simulink model "adaptiveBS"  (R2022a)
settings: Solver=VariableStepAuto  StartTime=0.0  StopTime=timeSpan  RelTol=1e-4
values from neighbouring files (symbols this model uses):
  K_d = 100 * eye(n)    [adaptiveBS_main.m]
  Lambda = 1 * eye(n)    [adaptiveBS_main.m]
  max_tau = 100 * [1 1 1 1 1 1]    [adaptiveBS_main.m]
  R = 10 * eye(n * 10)    [adaptiveBS_main.m]
undefined symbols (not defined in the file or in its folder): pi_est_0, pi_real
(part 5 of 5)

== matlab function adaptiveBS/Adattamento/MATLAB Function1 ==
  data: q input; Y output; dq input; ddq input
function Y = regressor(q, dq, ddq)

    % https://github.com/cdsousa/SymPyBotics

    %% Denavit-Hartenberg
    a2 = 0.4318;    a3 = 0.0203;
    d3 = 0.15005;   d4 = 0.4318;

    %% Variabili di giunto
    % q1 = q(1);  dq1 = dq(1);   ddq1 = ddq(1);
    % q2 = q(2);  dq2 = dq(2);   ddq2 = ddq(2);
    % q3 = q(3);  dq3 = dq(3);   ddq3 = ddq(3);
    % q4 = q(4);  dq4 = dq(4);   ddq4 = ddq(4);
    % q5 = q(5);  dq5 = dq(5);   ddq5 = ddq(5);
    % q6 = q(6);  dq6 = dq(6);   ddq6 = ddq(6);

    %% parms
    % (L_1xx, L_1xy, L_1xz, L_1yy, L_1yz, L_1zz, l_1x, l_1y, l_1z, m_1, L_2xx, L_2xy, L_2xz, L_2yy, L_2yz, L_2zz, l_2x, l_2y, l_2z, m_2, L_3xx, L_3xy, L_3xz, L_3yy, L_3yz, L_3zz, l_3x, l_3y, l_3z, m_3, L_4xx, L_4xy, L_4xz, L_4yy, L_4yz, L_4zz, l_4x, l_4y, l_4z, m_4, L_5xx, L_5xy, L_5xz, L_5yy, L_5yz, L_5zz, l_5x, l_5y, l_5z, m_5, L_6xx, L_6xy, L_6xz, L_6yy, L_6yz, L_6zz, l_6x, l_6y, l_6z, m_6)
    % Where:
    %   L is the link inertia tensor computed about the link frame;
    %   l is the link first moment of inertia;
    %   m is the link mass.
    % These are the so-called barycentric parameters, with respect to which the dynamic model is linear.


    x0 = sin(q(2));
    x1 = cos(q(2));
    x2 = dq(1) * x1;
    x3 = dq(2) * x2;
    x4 = ddq(1) * x0 + x3;
    x5 = dq(1) * x0;
    x6 = dq(2) * x5;
    x7 = -dq(2);
    x8 = x5 * x7;
    x9 = ddq(1) * x1;
    x10 = x8 + x9;
    x11 = x1 * (x3 + x4);
    x12 = ((dq(2)) * (dq(2)));
    x13 = ((x5) * (x5));
    x14 = -x13;
    x15 = x2 * x5;
    x16 = ddq(2) + x15;
    x17 = -x3;
    x18 = ((x2) * (x2));
    x19 = -x12;
    x20 = -x15;
    x21 = -a2;
    x22 = ((x0) * (x0)) * x21 + ((x1) * (x1)) * x21;
    x23 = a2 * dq(2);
    x24 = x23 * x5;
    x25 = x22 * x9 + x24;
    x26 = -x25;
    x27 = x24 + x25;
    x28 = -x18;
    x29 = x2 * x22;
    x30 = 9.81 * x0;
    x31 = a2 * ddq(2) + 9.81 * x1;
    x32 = sin(q(3));
    x33 = x10 * x32;
    x34 = cos(q(3));
    x35 = x34 * x4;
    x36 = x2 * x34;
    x37 = -x32;
    x38 = x37 * x5;
    x39 = x36 + x38;
    x40 = -dq(3);
    x41 = -x40;
    x42 = x33 + x35 + x39 * x41;
    x43 = x2 * x32;
    x44 = x34 * x5;
    x45 = x43 + x44;
    x46 = -x45;
    x47 = x40 + x7;
    x48 = x46 * x47;
    x49 = -ddq(2) - ddq(3);
    x50 = x39 * x45;
    x51 = -x50;
    x52 = x49 + x51;
    x53 = ((x45) * (x45));
    x54 = ((x47) * (x47));
    x55 = -x54;
    x56 = x53 + x55;
    x57 = x45 * x47;
    x58 = x10 * x34;
    x59 = x37 * x4;
    x60 = x40 * x45 + x58 + x59;
    x61 = x57 + x60;
    x62 = x34 * x61;
    x63 = x39 * x47;
    x64 = -x63;
    x65 = x42 + x64;
    x66 = x49 + x50;
    x67 = ((x39) * (x39));
    x68 = -x67;
    x69 = x54 + x68;
    x70 = x34 * x66;
    x71 = x55 + x68;
    x72 = -d3;
    x73 = x32 * x72;
    x74 = a3 * ((x32) * (x32)) + a3 * ((x34) * (x34));
    x75 = x37 * x74;
    x76 = dq(2) * x74 + x23 * x34 + x43 * x72 + x44 * x72;
    x77 = a3 * dq(3);
    x78 = x76 + x77;
    x79 = x26 + x46 * x77 + x58 * x74 + x59 * x74;
    x80 = d3 * x36 + x23 * x32;
    x81 = d3 * x38 + x80;
    x82 = x39 * x81;
    x83 = x46 * x78 + x79 + x82;
    x84 = x37 * x83;
    x85 = -x49;
    x86 = x50 + x85;
    x87 = x34 * x86;
    x88 = x1 * x22;
    x89 = x34 * x83;
    x90 = -x53;
    x91 = x68 + x90;
    x92 = x34 * x74;
    x93 = -x29;
    x94 = x36 * x74 + x38 * x74 + x93;
    x95 = x39 * x94;
    x96 = x47 * x78;
    x97 = d3 * x58 + x30 * x34 + x31 * x32 + x4 * x73 + x41 * x76 + x7 * x77;
    x98 = x95 - x96 - x97;
    x99 = x57 - x60;
    x100 = x42 + x63;
    x101 = a3 * ddq(3) + ddq(2) * x74 + x30 * x37 + x31 * x34 + x33 * x72 + x35 * x72 + x40 * (x5 * x73 + x80);
    x102 = x47 * x81;
    x103 = x101 - x102 + x45 * x94;
    x104 = x103 * x34;
    x105 = x100 * x34;
    x106 = x45 * x78 - x79 - x82;
    x107 = x55 + x90;
    x108 = -x42 + x63;
    x109 = x107 * x34;
    x110 = -x95 + x96 + x97;
    x111 = cos(q(4));
    x112 = sin(q(4));
    x113 = x112 * x49;
    x114 = x111 * x42;
    x115 = x112 * x45;
    x116 = x111 * x47;
    x117 = x115 - x116;
    x118 = -dq(4);
    x119 = x113 + x114 + x117 * x118;
    x120 = x112 * x47;
    x121 = x111 * x45;
    x122 = x120 + x121;
    x123 = dq(4) + x39;
    x124 = x122 * x123;
    x125 = -x124;
    x126 = x111 * x119 + x112 * x125;
    x127 = x117 * x122;
    x128 = x117 * x123;
    x129 = x119 + x128;
    x130 = ((x123) * (x123));
    x131 = -x130;
    x132 = ((x122) * (x122));
    x133 = x131 + x132;
    x134 = -x117;
    x135 = x122 * x134;
    x136 = ddq(4) + x60;
    x137 = x135 + x136;
    x138 = x111 * x137 + x112 * x133;
    x139 = -x111;
    x140 = x112 * x42;
    x141 = dq(4) * x122 + x139 * x49 + x140;
    x142 = x124 + x141;
    x143 = x123 * x134;
    x144 = x119 + x143;
    x145 = x111 * x142 + x112 * x144;
    x146 = -x132;
    x147 = ((x117) * (x117));
    x148 = x146 + x147;
    x149 = x111 * x143 + x112 * x124;
    x150 = x127 + x136;
    x151 = x112 * x150;
    x152 = -x147;
    x153 = x130 + x152;
    x154 = x111 * x153 + x151;
    x155 = x125 + x141;
    x156 = x111 * x128 + x112 * x141;
    x157 = x127 - x136;
    x158 = d4 * x111;
    x159 = -d4;
    x160 = d4 * x116 + x111 * x81 + x112 * x94 + x115 * x159;
    x161 = d4 * x120 + d4 * x121 + x112 * x81 + x139 * x94;
    x162 = -x161;
    x163 = x101 + x117 * x160 + x122 * x162;
    x164 = x131 + x152;
    x165 = x112 * x164;
    x166 = x112 * x163 + x157 * x158 + x159 * x165;
    x167 = x142 * x34;
    x168 = x139 * x157 + x165;
    x169 = x112 * x157;
    x170 = x111 * x164 + x169;
    x171 = x123 * x160;
    x172 = x122 * x78;
    x173 = d4 * x113 + d4 * x114 + dq(4) * x160 + x112 * x97 + x139 * x79;
    x174 = -x173;
    x175 = x171 - x172 + x174;
    x176 = -x141;
    x177 = x124 + x176;
    x178 = x112 * x177;
    x179 = x129 * x139 + x178;
    x180 = x146 + x152;
    x181 = x180 * x34;
    x182 = x112 * x129;
    x183 = x111 * x177 + x182;
    x184 = x111 * x97 + x112 * x79 + x118 * x161 + x140 * x159 + x158 * x49;
    x185 = x117 * x78 + x123 * x162 - x184;
    x186 = -x171 + x172 + x173;
    x187 = x111 * x186 + x112 * x185 + x129 * x158 + x159 * x178;
    x188 = x131 + x146;
    x189 = x139 * x188 + x151;
    x190 = -x119 + x128;
    x191 = x190 * x34;
    x192 = x123 * x161 + x134 * x78 + x184;
    x193 = x112 * x188;
    x194 = x111 * x150 + x193;
    x195 = -x101;
    x196 = x122 * x161 + x134 * x160 + x195;
    x197 = x111 * x196 + x151 * x159 + x158 * x188;
    x198 = x112 * x192;
    x199 = x139 * x186 + x198;
    x200 = x112 * x186;
    x201 = x111 * x192 + x200;
    x202 = x158 * x186 + x159 * x198;
    x203 = x163 * x34;
    x204 = sin(q(5));
    x205 = cos(q(5));
    x206 = x122 * x205 + x123 * x204;
    x207 = -dq(5);
    x208 = x134 + x207;
    x209 = x206 * x208;
    x210 = -x209;
    x211 = -x204;
    x212 = x122 * x211 + x123 * x205;
    x213 = -x207;
    x214 = x119 * x205 + x136 * x204 + x212 * x213;
    x215 = x204 * x214 + x205 * x210;
    x216 = x205 * x214 + x210 * x211;
    x217 = x206 * x212;
    x218 = -x217;
    x219 = x111 * x216 + x112 * x218;
    x220 = x208 * x212;
    x221 = x214 + x220;
    x222 = -x221;
    x223 = -ddq(5) + x176;
    x224 = x218 + x223;
    x225 = ((x206) * (x206));
    x226 = ((x208) * (x208));
    x227 = -x226;
    x228 = x225 + x227;
    x229 = x205 * x224 + x211 * x228;
    x230 = x111 * x229 + x112 * x222;
    x231 = x204 * x224 + x205 * x228;
    x232 = -x225;
    x233 = ((x212) * (x212));
    x234 = -x232 - x233;
    x235 = -x220;
    x236 = x214 + x235;
    x237 = x119 * x211 + x136 * x205 + x206 * x207;
    x238 = x209 + x237;
    x239 = x205 * x238 + x211 * x236;
    x240 = x111 * x239 + x112 * x234;
    x241 = x204 * x238 + x205 * x236;
    x242 = -x223;
    x243 = x205 * x235 + x209 * x211;
    x244 = x111 * x243 + x112 * x242;
    x245 = x204 * x235 + x205 * x209;
    x246 = x217 + x223;
    x247 = -x233;
    x248 = x226 + x247;
    x249 = x205 * x248 + x211 * x246;
    x250 = -x210 - x237;
    x251 = x111 * x249 + x112 * x250;
    x252 = x205 * x246;
    x253 = x204 * x248 + x252;
    x254 = x204 * x220 + x205 * x237;
    x255 = x205 * x220 + x211 * x237;
    x256 = -x218;
    x257 = x111 * x255 + x112 * x256;
    x258 = -x238;
    x259 = x112 * x258;
    x260 = x217 + x242;
    x261 = x227 + x247;
    x262 = x205 * x261 + x211 * x260;
    x263 = x111 * x262 + x259;
    x264 = x204 * x261 + x205 * x260;
    x265 = x264 * x34;
    x266 = -x206;
    x267 = x160 * x211 + x205 * x78;
    x268 = x160 * x205 + x204 * x78;
    x269 = x212 * x268;
    x270 = x174 + x266 * x267 + x269;
    x271 = x205 * x270;
    x272 = x211 * x270;
    x273 = x112 * x262;
    x274 = x208 * x268;
    x275 = x101 * x205 + x184 * x211 + x207 * x268;
    x276 = -x275;
    x277 = -x162 * x266 - x274 - x276;
    x278 = x111 * x272 + x112 * x277 + x158 * x258 + x159 * x273;
    x279 = x139 * x258 + x273;
    x280 = x209 - x237;
    x281 = x205 * x280 + x211 * x221;
    x282 = x112 * x281;
    x283 = -x232 - x247;
    x284 = x139 * x283 + x282;
    x285 = x162 * x206 - x274 + x275;
    x286 = x205 * x285;
    x287 = x162 * x212;
    x288 = x208 * x267;
    x289 = x101 * x204 + x184 * x205 + x213 * x267;
    x290 = x287 - x288 - x289;
    x291 = x211 * x290 + x286;
    x292 = x111 * x291 + x158 * x283 + x159 * x282;
    x293 = x204 * x285 + x205 * x290;
    x294 = x204 * x280 + x205 * x221;
    x295 = x294 * x34;
    x296 = x112 * x283;
    x297 = x111 * x281 + x296;
    x298 = x227 + x232;
    x299 = x204 * x246 + x205 * x298;
    x300 = x299 * x34;
    x301 = -x287 + x288 + x289;
    x302 = -x301;
    x303 = x211 * x298 + x252;
    x304 = x112 * x303;
    x305 = x214 - x220;
    x306 = -x174 + x206 * x267 - x269;
    x307 = x205 * x306;
    x308 = x111 * x307 + x112 * x302 + x158 * x305 + x159 * x304;
    x309 = x139 * x305 + x304;
    x310 = x204 * x306;
    x311 = x112 * x305;
    x312 = x111 * x303 + x311;
    x313 = x205 * x301 + x211 * x285;
    x314 = x112 * x313;
    x315 = -x270;
    x316 = x158 * x315 + x159 * x314;
    x317 = x139 * x315 + x314;
    x318 = x112 * x315;
    x319 = x111 * x313 + x318;
    x320 = x204 * x301 + x286;
    x321 = x320 * x34;
    x322 = sin(q(6));
    x323 = cos(q(6));
    x324 = x206 * x323 + x208 * x322;
    x325 = dq(6) + x212;
    x326 = x324 * x325;
    x327 = -x322;
    x328 = x206 * x327 + x208 * x323;
    x329 = dq(6) * x328 + x214 * x323 + x223 * x322;
    x330 = x323 * x329 + x326 * x327;
    x331 = x324 * x328;
    x332 = -x331;
    x333 = x205 * x330 + x211 * x332;
    x334 = -x322 * x329 - x323 * x326;
    x335 = x111 * x333 + x112 * x334;
    x336 = x204 * x330 + x205 * x332;
    x337 = x325 * x328;
    x338 = x329 + x337;
    x339 = -x326;
    x340 = -dq(6);
    x341 = x214 * x327 + x223 * x323 + x324 * x340;
    x342 = x339 + x341;
    x343 = x323 * x342 + x327 * x338;
    x344 = ((x328) * (x328));
    x345 = -x344;
    x346 = ((x324) * (x324));
    x347 = x345 + x346;
    x348 = x204 * x343 + x205 * x347;
    x349 = x205 * x343 + x211 * x347;
    x350 = -x322 * x342 - x323 * x338;
    x351 = x111 * x349 + x112 * x350;
    x352 = -x337;
    x353 = x329 + x352;
    x354 = ((x325) * (x325));
    x355 = -x346;
    x356 = x354 + x355;
    x357 = ddq(6) + x237;
    x358 = x331 + x357;
    x359 = x323 * x358;
    x360 = x327 * x356 + x359;
    x361 = x204 * x360 + x205 * x353;
    x362 = x205 * x360 + x211 * x353;
    x363 = -x322 * x358 - x323 * x356;
    x364 = x111 * x362 + x112 * x363;
    x365 = x323 * x352 + x327 * x341;
    x366 = x205 * x365 + x211 * x331;
    x367 = -x322 * x352 - x323 * x341;
    x368 = x111 * x366 + x112 * x367;
    x369 = x204 * x365 + x205 * x331;
    x370 = x326 + x341;
    x371 = -x354;
    x372 = x344 + x371;
    x373 = x332 + x357;
    x374 = x323 * x372 + x327 * x373;
    x375 = x205 * x374 + x211 * x370;
    x376 = -x322 * x372 - x323 * x373;
    x377 = x111 * x375 + x112 * x376;
    x378 = x204 * x374 + x205 * x370;
    x379 = x323 * x337 + x327 * x339;
    x380 = x204 * x379 + x205 * x357;
    x381 = x205 * x379 + x211 * x357;
    x382 = -x322 * x337 - x323 * x339;
    x383 = x111 * x381 + x112 * x382;
    x384 = x345 + x371;
    x385 = x323 * x384 + x327 * x358;
    x386 = x326 - x341;
    x387 = x204 * x385 + x205 * x386;
    x388 = x34 * x387;
    x389 = -x322 * x384 - x359;
    x390 = x205 * x385 + x211 * x386;
    x391 = x112 * x390;
    x392 = -x324;
    x393 = x162 * x323 + x268 * x327;
    x394 = x162 * x322 + x268 * x323;
    x395 = x328 * x394;
    x396 = x276 + x392 * x393 + x395;
    x397 = -x323 * x396;
    x398 = x174 * x323 + x289 * x327 + x340 * x394;
    x399 = x325 * x394;
    x400 = x267 * x392 + x398 + x399;
    x401 = x327 * x396;
    x402 = x205 * x401 + x211 * x400;
    x403 = x111 * x402 + x112 * x397 + x158 * x389 + x159 * x391;
    x404 = x139 * x389 + x391;
    x405 = x112 * x389;
    x406 = x111 * x390 + x405;
    x407 = x204 * x401 + x205 * x400;
    x408 = x325 * x393;
    x409 = x267 * x328;
    x410 = dq(6) * x393 + x174 * x322 + x289 * x323;
    x411 = x408 - x409 - x410;
    x412 = x275 + x324 * x393 - x395;
    x413 = x323 * x412;
    x414 = x204 * x413 + x205 * x411;
    x415 = x355 + x371;
    x416 = x331 - x357;
    x417 = x323 * x416 + x327 * x415;
    x418 = x204 * x417 + x205 * x338;
    x419 = -x322 * x416 - x323 * x415;
    x420 = x112 * x419;
    x421 = x205 * x417 + x211 * x338;
    x422 = x111 * x421 + x420;
    x423 = x112 * x421;
    x424 = x139 * x419 + x423;
    x425 = -x322 * x412;
    x426 = x205 * x413 + x211 * x411;
    x427 = x111 * x426 + x112 * x425 + x158 * x419 + x159 * x423;
    x428 = x34 * x418;
    x429 = -x329 + x337;
    x430 = -x322 * x370 - x323 * x429;
    x431 = x345 + x355;
    x432 = x323 * x370 + x327 * x429;
    x433 = x205 * x432 + x211 * x431;
    x434 = x112 * x433;
    x435 = x139 * x430 + x434;
    x436 = x267 * x324 - x398 - x399;
    x437 = -x408 + x409 + x410;
    x438 = x323 * x437;
    x439 = -x322 * x436 - x438;
    x440 = x323 * x436 + x327 * x437;
    x441 = x205 * x440;
    x442 = x111 * x441 + x112 * x439 + x158 * x430 + x159 * x434;
    x443 = x204 * x432 + x205 * x431;
    x444 = x112 * x430;
    x445 = x111 * x433 + x444;
    x446 = x204 * x440;
    x447 = x34 * x443;
    x448 = -x322 * x437 - x323 * x400;
    x449 = x327 * x400 + x438;
    x450 = x205 * x449 + x211 * x412;
    x451 = x112 * x450;
    x452 = x158 * x448 + x159 * x451;
    x453 = x204 * x449 + x205 * x412;
    x454 = x139 * x448 + x451;
    x455 = x112 * x448;
    x456 = x111 * x450 + x455;
    x457 = x34 * x453;
    x458 = x31 + x5 * x93;
    x459 = -x100;
    x460 = -x67 - x90;
    x461 = -x48 - x60;
    x462 = -x51;
    x463 = -x102 - x195 - x46 * x94;
    x464 = -x110;
    x465 = -x112 * x119 - x125 * x139;
    x466 = -x112 * x137 - x133 * x139;
    x467 = -x112 * x142 - x139 * x144;
    x468 = -x112 * x143 - x124 * x139;
    x469 = -x112 * x153 - x139 * x150;
    x470 = -x112 * x128 - x139 * x141;
    x471 = -d4 * x169 - x139 * x163 - x158 * x164;
    x472 = -d4 * x182 - x139 * x185 - x158 * x177 - x200;
    x473 = -d4 * x193 - x112 * x196 - x150 * x158;
    x474 = -d4 * x200 - x158 * x192;
    x475 = -x112 * x216 - x139 * x218;
    x476 = -x112 * x229 - x139 * x222;
    x477 = -x112 * x239 - x139 * x234;
    x478 = -x112 * x243 - x139 * x242;
    x479 = -x112 * x249 - x139 * x250;
    x480 = -x112 * x255 - x139 * x256;
    x481 = -d4 * x259 - x112 * x272 - x139 * x277 - x158 * x262;
    x482 = -d4 * x296 - x112 * x291 - x158 * x281;
    x483 = -d4 * x311 - x112 * x307 - x139 * x302 - x158 * x303;
    x484 = -d4 * x318 - x158 * x313;
    x485 = -x112 * x333 - x139 * x334;
    x486 = -x112 * x349 - x139 * x350;
    x487 = -x112 * x362 - x139 * x363;
    x488 = -x112 * x366 - x139 * x367;
    x489 = -x112 * x375 - x139 * x376;
    x490 = -x112 * x381 - x139 * x382;
    x491 = -d4 * x405 - x112 * x402 - x139 * x397 - x158 * x390;
    x492 = -d4 * x420 - x112 * x426 - x139 * x425 - x158 * x421;
    x493 = -d4 * x444 - x112 * x441 - x139 * x439 - x158 * x433;
    x494 = -d4 * x455 - x158 * x450;

    
    n = 6;
    H = zeros(n * n * 10, 1); % = 360       Y = 6 * 60

    H(1) = 0;
    H(2) = 0;
    H(3) = 0;
    H(4) = ddq(1);
    H(5) = 0;
    H(6) = 0;
    H(7) = 0;
    H(8) = 0;
    H(9) = 0;
    H(10) = 0;
    H(11) = x0 * x4 + x1 * x6;
    H(12) = x0 * (x10 + x8) + x11;
    H(13) = x0 * x16 + x1 * (x12 + x14);
    H(14) = x0 * x17 + x1 * x10;
    H(15) = x0 * (x18 + x19) + x1 * (ddq(2) + x20);
    H(16) = x0 * x3 + x1 * x8;
    H(17) = x1 * x22 * (-x10 + x6) + x1 * (-x24 + x26);
    H(18) = x0 * x27 + x11 * x22;
    H(19) = x0 * (x29 * x5 - x31) + x1 * x22 * (x14 + x28) + x1 * (x2 * x29 + x23 * x7 + x30);
    H(20) = x1 * x22 * x27;
    H(21) = x0 * (x34 * x42 + x37 * x48) + x1 * (x32 * x42 + x34 * x48);
    H(22) = x0 * (x34 * x52 + x37 * x56) + x1 * (x32 * x52 + x34 * x56);
    H(23) = x0 * (x37 * x65 + x62) + x1 * (x32 * x61 + x34 * x65);
    H(24) = x0 * (x34 * x64 + x37 * x57) + x1 * (x32 * x64 + x34 * x57);
    H(25) = x0 * (x34 * x69 + x37 * x66) + x1 * (x32 * x69 + x70);
    H(26) = x0 * (x34 * x63 + x37 * x60) + x1 * (x32 * x63 + x34 * x60);
    H(27) = x0 * (x61 * x75 + x71 * x73 + x72 * x87 + x84) + x1 * (d3 * x34 * x71 + x62 * x74 + x73 * x86 + x89) - x61 * x88;
    H(28) = x0 * (x104 + x105 * x72 + x37 * x98 + x73 * x99 + x75 * x91) + x1 * (d3 * x34 * x99 + x100 * x73 + x103 * x32 + x34 * x98 + x91 * x92) - x88 * x91;
    H(29) = x0 * (x106 * x34 + x108 * x75 + x109 * x72 + x66 * x73) + x1 * (d3 * x70 + x106 * x32 + x107 * x73 + x108 * x92) - x108 * x88;
    H(30) = x0 * (x104 * x72 + x110 * x73 + x74 * x84) + x1 * (d3 * x110 * x34 + x103 * x73 + x74 * x89) - x83 * x88;
    H(31) = x0 * (x126 * x34 + x127 * x37) + x1 * (x126 * x32 + x127 * x34);
    H(32) = x0 * (x129 * x37 + x138 * x34) + x1 * (x129 * x34 + x138 * x32);
    H(33) = x0 * (x145 * x34 + x148 * x37) + x1 * (x145 * x32 + x148 * x34);
    H(34) = x0 * (x136 * x37 + x149 * x34) + x1 * (x136 * x34 + x149 * x32);
    H(35) = x0 * (x154 * x34 + x155 * x37) + x1 * (x154 * x32 + x155 * x34);
    H(36) = x0 * (x135 * x37 + x156 * x34) + x1 * (x135 * x34 + x156 * x32);
    H(37) = x0 * (x166 * x34 + x167 * x72 + x168 * x75 + x170 * x73 + x175 * x37) + x1 * (d3 * x170 * x34 + x142 * x73 + x166 * x32 + x168 * x92 + x175 * x34) - x168 * x88;
    H(38) = x0 * (x179 * x75 + x181 * x72 + x183 * x73 + x187 * x34) + x1 * (d3 * x183 * x34 + x179 * x92 + x180 * x73 + x187 * x32) - x179 * x88;
    H(39) = x0 * (x189 * x75 + x191 * x72 + x192 * x37 + x194 * x73 + x197 * x34) + x1 * (d3 * x194 * x34 + x189 * x92 + x190 * x73 + x192 * x34 + x197 * x32) - x189 * x88;
    H(40) = x0 * (x199 * x75 + x201 * x73 + x202 * x34 + x203 * x72) + x1 * (d3 * x201 * x34 + x163 * x73 + x199 * x92 + x202 * x32) - x199 * x88;
    H(41) = x0 * (x215 * x37 + x219 * x34) + x1 * (x215 * x34 + x219 * x32);
    H(42) = x0 * (x230 * x34 + x231 * x37) + x1 * (x230 * x32 + x231 * x34);
    H(43) = x0 * (x240 * x34 + x241 * x37) + x1 * (x240 * x32 + x241 * x34);
    H(44) = x0 * (x244 * x34 + x245 * x37) + x1 * (x244 * x32 + x245 * x34);
    H(45) = x0 * (x251 * x34 + x253 * x37) + x1 * (x251 * x32 + x253 * x34);
    H(46) = x0 * (x254 * x37 + x257 * x34) + x1 * (x254 * x34 + x257 * x32);
    H(47) = x0 * (x263 * x73 + x265 * x72 + x271 * x37 + x278 * x34 + x279 * x75) + x1 * (d3 * x263 * x34 + x264 * x73 + x271 * x34 + x278 * x32 + x279 * x92) - x279 * x88;
    H(48) = x0 * (x284 * x75 + x292 * x34 + x293 * x37 + x295 * x72 + x297 * x73) + x1 * (d3 * x297 * x34 + x284 * x92 + x292 * x32 + x293 * x34 + x294 * x73) - x284 * x88;
    H(49) = x0 * (x300 * x72 + x308 * x34 + x309 * x75 + x310 * x37 + x312 * x73) + x1 * (d3 * x312 * x34 + x299 * x73 + x308 * x32 + x309 * x92 + x310 * x34) - x309 * x88;
    H(50) = x0 * (x316 * x34 + x317 * x75 + x319 * x73 + x321 * x72) + x1 * (d3 * x319 * x34 + x316 * x32 + x317 * x92 + x320 * x73) - x317 * x88;
    H(51) = x0 * (x335 * x34 + x336 * x37) + x1 * (x32 * x335 + x336 * x34);
    H(52) = x0 * (x34 * x351 + x348 * x37) + x1 * (x32 * x351 + x34 * x348);
    H(53) = x0 * (x34 * x364 + x361 * x37) + x1 * (x32 * x364 + x34 * x361);
    H(54) = x0 * (x34 * x368 + x369 * x37) + x1 * (x32 * x368 + x34 * x369);
    H(55) = x0 * (x34 * x377 + x37 * x378) + x1 * (x32 * x377 + x34 * x378);
    H(56) = x0 * (x34 * x383 + x37 * x380) + x1 * (x32 * x383 + x34 * x380);
    H(57) = x0 * (x34 * x403 + x37 * x407 + x388 * x72 + x404 * x75 + x406 * x73) + x1 * (d3 * x34 * x406 + x32 * x403 + x34 * x407 + x387 * x73 + x404 * x92) - x404 * x88;
    H(58) = x0 * (x34 * x427 + x37 * x414 + x422 * x73 + x424 * x75 + x428 * x72) + x1 * (d3 * x34 * x422 + x32 * x427 + x34 * x414 + x418 * x73 + x424 * x92) - x424 * x88;
    H(59) = x0 * (x34 * x442 + x37 * x446 + x435 * x75 + x445 * x73 + x447 * x72) + x1 * (d3 * x34 * x445 + x32 * x442 + x34 * x446 + x435 * x92 + x443 * x73) - x435 * x88;
    H(60) = x0 * (x34 * x452 + x454 * x75 + x456 * x73 + x457 * x72) + x1 * (d3 * x34 * x456 + x32 * x452 + x453 * x73 + x454 * x92) - x454 * x88;
    H(61) = 0;
    H(62) = 0;
    H(63) = 0;
    H(64) = 0;
    H(65) = 0;
    H(66) = 0;
    H(67) = 0;
    H(68) = 0;
    H(69) = 0;
    H(70) = 0;
    H(71) = x20;
    H(72) = x13 + x28;
    H(73) = x17 + x4;
    H(74) = x15;
    H(75) = x10 + x6;
    H(76) = ddq(2);
    H(77) = a2 * x16 + x458;
    H(78) = a2 * (x14 + x19) + dq(2) * x23 + x2 * x93 - x30;
    H(79) = a2 * (x3 - x4);
    H(80) = a2 * x458;
    H(81) = x51;
    H(82) = x459;
    H(83) = x460;
    H(84) = x85;
    H(85) = x461;
    H(86) = x462;
    H(87) = a2 * (x32 * x71 + x87) + x463 + x74 * x86;
    H(88) = a2 * (x105 + x32 * x99) + x100 * x74;
    H(89) = a2 * (x109 + x32 * x66) + x107 * x74 + x464;
    H(90) = a2 * (x104 + x110 * x32) + x103 * x74;
    H(91) = x465;
    H(92) = x466;
    H(93) = x467;
    H(94) = x468;
    H(95) = x469;
    H(96) = x470;
    H(97) = a2 * (x167 + x170 * x32) + x142 * x74 + x471;
    H(98) = a2 * (x181 + x183 * x32) + x180 * x74 + x472;
    H(99) = a2 * (x191 + x194 * x32) + x190 * x74 + x473;
    H(100) = a2 * (x201 * x32 + x203) + x163 * x74 + x474;
    H(101) = x475;
    H(102) = x476;
    H(103) = x477;
    H(104) = x478;
    H(105) = x479;
    H(106) = x480;
    H(107) = a2 * (x263 * x32 + x265) + x264 * x74 + x481;
    H(108) = a2 * (x295 + x297 * x32) + x294 * x74 + x482;
    H(109) = a2 * (x300 + x312 * x32) + x299 * x74 + x483;
    H(110) = a2 * (x319 * x32 + x321) + x320 * x74 + x484;
    H(111) = x485;
    H(112) = x486;
    H(113) = x487;
    H(114) = x488;
    H(115) = x489;
    H(116) = x490;
    H(117) = a2 * (x32 * x406 + x388) + x387 * x74 + x491;
    H(118) = a2 * (x32 * x422 + x428) + x418 * x74 + x492;
    H(119) = a2 * (x32 * x445 + x447) + x443 * x74 + x493;
    H(120) = a2 * (x32 * x456 + x457) + x453 * x74 + x494;
    H(121) = 0;
    H(122) = 0;
    H(123) = 0;
    H(124) = 0;
    H(125) = 0;
    H(126) = 0;
    H(127) = 0;
    H(128) = 0;
    H(129) = 0;
    H(130) = 0;
    H(131) = 0;
    H(132) = 0;
    H(133) = 0;
    H(134) = 0;
    H(135) = 0;
    H(136) = 0;
    H(137) = 0;
    H(138) = 0;
    H(139) = 0;
    H(140) = 0;
    H(141) = x51;
    H(142) = x459;
    H(143) = x460;
    H(144) = x85;
    H(145) = x461;
    H(146) = x462;
    H(147) = a3 * x86 + x463;
    H(148) = a3 * x100;
    H(149) = a3 * x107 + x464;
    H(150) = a3 * x103;
    H(151) = x465;
    H(152) = x466;
    H(153) = x467;
    H(154) = x468;
    H(155) = x469;
    H(156) = x470;
    H(157) = a3 * x142 + x471;
    H(158) = a3 * x180 + x472;
    H(159) = a3 * x190 + x473;
    H(160) = a3 * x163 + x474;
    H(161) = x475;
    H(162) = x476;
    H(163) = x477;
    H(164) = x478;
    H(165) = x479;
    H(166) = x480;
    H(167) = a3 * x264 + x481;
    H(168) = a3 * x294 + x482;
    H(169) = a3 * x299 + x483;
    H(170) = a3 * x320 + x484;
    H(171) = x485;
    H(172) = x486;
    H(173) = x487;
    H(174) = x488;
    H(175) = x489;
    H(176) = x490;
    H(177) = a3 * x387 + x491;
    H(178) = a3 * x418 + x492;
    H(179) = a3 * x443 + x493;
    H(180) = a3 * x453 + x494;
    H(181) = 0;
    H(182) = 0;
    H(183) = 0;
    H(184) = 0;
    H(185) = 0;
    H(186) = 0;
    H(187) = 0;
    H(188) = 0;
    H(189) = 0;
    H(190) = 0;
    H(191) = 0;
    H(192) = 0;
    H(193) = 0;
    H(194) = 0;
    H(195) = 0;
    H(196) = 0;
    H(197) = 0;
    H(198) = 0;
    H(199) = 0;
    H(200) = 0;
    H(201) = 0;
    H(202) = 0;
    H(203) = 0;
    H(204) = 0;
    H(205) = 0;
    H(206) = 0;
    H(207) = 0;
    H(208) = 0;
    H(209) = 0;
    H(210) = 0;
    H(211) = x127;
    H(212) = x129;
    H(213) = x148;
    H(214) = x136;
    H(215) = x155;
    H(216) = x135;
    H(217) = x175;
    H(218) = 0;
    H(219) = x192;
    H(220) = 0;
    H(221) = x215;
    H(222) = x231;
    H(223) = x241;
    H(224) = x245;
    H(225) = x253;
    H(226) = x254;
    H(227) = x271;
    H(228) = x293;
    H(229) = x310;
    H(230) = 0;
    H(231) = x336;
    H(232) = x348;
    H(233) = x361;
    H(234) = x369;
    H(235) = x378;
    H(236) = x380;
    H(237) = x407;
    H(238) = x414;
    H(239) = x446;
    H(240) = 0;
    H(241) = 0;
    H(242) = 0;
    H(243) = 0;
    H(244) = 0;
    H(245) = 0;
    H(246) = 0;
    H(247) = 0;
    H(248) = 0;
    H(249) = 0;
    H(250) = 0;
    H(251) = 0;
    H(252) = 0;
    H(253) = 0;
    H(254) = 0;
    H(255) = 0;
    H(256) = 0;
    H(257) = 0;
    H(258) = 0;
    H(259) = 0;
    H(260) = 0;
    H(261) = 0;
    H(262) = 0;
    H(263) = 0;
    H(264) = 0;
    H(265) = 0;
    H(266) = 0;
    H(267) = 0;
    H(268) = 0;
    H(269) = 0;
    H(270) = 0;
    H(271) = 0;
    H(272) = 0;
    H(273) = 0;
    H(274) = 0;
    H(275) = 0;
    H(276) = 0;
    H(277) = 0;
    H(278) = 0;
    H(279) = 0;
    H(280) = 0;
    H(281) = x218;
    H(282) = x222;
    H(283) = x234;
    H(284) = x242;
    H(285) = x250;
    H(286) = x256;
    H(287) = x277;
    H(288) = 0;
    H(289) = x302;
    H(290) = 0;
    H(291) = x334;
    H(292) = x350;
    H(293) = x363;
    H(294) = x367;
    H(295) = x376;
    H(296) = x382;
    H(297) = x397;
    H(298) = x425;
    H(299) = x439;
    H(300) = 0;
    H(301) = 0;
    H(302) = 0;
    H(303) = 0;
    H(304) = 0;
    H(305) = 0;
    H(306) = 0;
    H(307) = 0;
    H(308) = 0;
    H(309) = 0;
    H(310) = 0;
    H(311) = 0;
    H(312) = 0;
    H(313) = 0;
    H(314) = 0;
    H(315) = 0;
    H(316) = 0;
    H(317) = 0;
    H(318) = 0;
    H(319) = 0;
    H(320) = 0;
    H(321) = 0;
    H(322) = 0;
    H(323) = 0;
    H(324) = 0;
    H(325) = 0;
    H(326) = 0;
    H(327) = 0;
    H(328) = 0;
    H(329) = 0;
    H(330) = 0;
    H(331) = 0;
    H(332) = 0;
    H(333) = 0;
    H(334) = 0;
    H(335) = 0;
    H(336) = 0;
    H(337) = 0;
    H(338) = 0;
    H(339) = 0;
    H(340) = 0;
    H(341) = 0;
    H(342) = 0;
    H(343) = 0;
    H(344) = 0;
    H(345) = 0;
    H(346) = 0;
    H(347) = 0;
    H(348) = 0;
    H(349) = 0;
    H(350) = 0;
    H(351) = x332;
    H(352) = x347;
    H(353) = x353;
    H(354) = x331;
    H(355) = x370;
    H(356) = x357;
    H(357) = x400;
    H(358) = x411;
    H(359) = 0;
    H(360) = 0;


    Y = reshape(H,60,6)';


end

== matlab function adaptiveBS/Adattamento/MATLAB Function ==
  data: R input; Y input; dpi_h output; s input
function dpi_h = dpiHat(R, Y, s)

dpi_h = R \ transpose(Y) * s;

end
